simulink model "AntilockBraking"  (R2020b)
settings: Solver=VariableStepAuto  StartTime=0.0  StopTime=10.0  RelTol=1e-3
model workspace (MAT data in the model file):
  I = 5
  Kf = 1
  PBmax = 1500
  Rr = 1.25
  TB = 0.01
  ctrl = 1
  g = 32.18
  h : matlab.ui.Figure (value not decoded)
  m = 50
  mu = [0 0.4 0.8 0.97 1 0.98 0.96 0.94 0.92 0.9 0.88 0.855 0.83 0.81 0.79 0.77 0.75 0.73 0.72 0.71 0.7]
  out = Simulink.SimulationOutput
  out.Data.tout = [0; 0.2; 0.4; 0.6; 0.8; 1; 1.2; 1.4; 1.6; 1.8; 2; 2.2; 2.4; 2.6; 2.8; 3; 3.2; 3.4; 3.6; 3.8; 4; 4.2; 4.4; 4.6; 4.8; 5; 5.2; 5.4; 5.6; 5.8; 6; 6.2; 6.4; 6.6; 6.8; 7; 7.2; 7.4; 7.6; 7.8; 8; 8.2; 8.4; 8.6; 8.8; 9; 9.2; 9.4; 9.6; 9.8; 10]
  out.Data.yout = Simulink.SimulationData.Dataset
  out.Data.yout.any.Name = 'yout'
  out.Data.yout.any.Version = 3
  out.Data.yout.any.Storage = Simulink.SimulationData.Storage.RamDatasetStorage
  out.Data.yout.any.Storage.any.Version = 2
  out.Data.yout.any.Storage.any.Elements{1} = Simulink.SimulationData.Signal
  out.Data.yout.any.Storage.any.Elements{1}.Version = 1
  out.Data.yout.any.Storage.any.Elements{1}.BlockPath = Simulink.SimulationData.BlockPath
  out.Data.yout.any.Storage.any.Elements{1}.BlockPath.path = {'AntilockBraking/Outport1'}
  out.Data.yout.any.Storage.any.Elements{1}.Values = timeseries
  out.Data.yout.any.Storage.any.Elements{1}.Values.Name = 'Ww'
  out.Data.yout.any.Storage.any.Elements{1}.Values.DataInfo = tsdata.datametadata
  out.Data.yout.any.Storage.any.Elements{1}.Values.DataInfo.Interpolation = tsdata.interpolation
  out.Data.yout.any.Storage.any.Elements{1}.Values.DataInfo.Interpolation.Fhandle : function handle (value not decoded)
  out.Data.yout.any.Storage.any.Elements{1}.Values.DataInfo.Interpolation.Name = 'linear'
  out.Data.yout.any.Storage.any.Elements{1}.Values.TimeInfo = tsdata.timemetadata
  out.Data.yout.any.Storage.any.Elements{1}.Values.TimeInfo.Length = 51
  out.Data.yout.any.Storage.any.Elements{1}.Values.TimeInfo.DuplicateTimes = 0
  out.Data.yout.any.Storage.any.Elements{1}.Values.TimeInfo.Time_ = [0; 0.2; 0.4; 0.6; 0.8; 1; 1.2; 1.4; 1.6; 1.8; 2; 2.2; 2.4; 2.6; 2.8; 3; 3.2; 3.4; 3.6; 3.8; 4; 4.2; 4.4; 4.6; 4.8; 5; 5.2; 5.4; 5.6; 5.8; 6; 6.2; 6.4; 6.6; 6.8; 7; 7.2; 7.4; 7.6; 7.8; 8; 8.2; 8.4; 8.6; 8.8; 9; 9.2; 9.4; 9.6; 9.8; 10]
  out.Data.yout.any.Storage.any.Elements{1}.Values.TimeInfo.Initialized = 1
  out.Data.yout.any.Storage.any.Elements{1}.Values.QualityInfo = tsdata.qualmetadata
  out.Data.yout.any.Storage.any.Elements{1}.Values.Data_ = [70.4; 70.4; 70.4; 70.4; 70.4; 70.4; 70.4; 70.4; 70.4; 70.4; 70.4; 70.4; 70.4; 70.4; 70.4; 70.4; 70.4; 70.4; 70.4; 70.4; 70.4; 70.4; 70.4; 70.4; 70.4; 70.4; 70.4; 70.4; 70.4; 70.4; 70.4; 70.4; 70.4; 70.4; 70.4; 70.4; 70.4; 70.4; 70.4; 70.4; 70.4; 70.4; 70.4; 70.4; 70.4; 70.4; 70.4; 70.4; 70.4; 70.4; 70.4]
  out.Data.yout.any.Storage.any.Elements{1}.Name = 'Ww'
  out.Metadata = Simulink.SimulationMetadata
  out.Metadata.ModelInfo.ModelName = 'AntilockBraking'
  out.Metadata.ModelInfo.ModelVersion = '1.2'
  out.Metadata.ModelInfo.ModelFilePath = 'C:\Users\baner\MATLAB\Projects\Problem_3_AntilockBrakingSystem\AntilockBraking.slx'
  out.Metadata.ModelInfo.UserID = 'baner'
  out.Metadata.ModelInfo.MachineName = 'LAPTOP-PBLSD5RN'
  out.Metadata.ModelInfo.Platform = 'PCWIN64'
  out.Metadata.ModelInfo.ModelStructuralChecksum = [3722489804; 3647447735; 815880221; 3047452302]
  out.Metadata.ModelInfo.SimulationMode = 'normal'
  out.Metadata.ModelInfo.StartTime = 0
  out.Metadata.ModelInfo.StopTime = 10
  out.Metadata.ModelInfo.SolverInfo.Type = 'Variable-Step'
  out.Metadata.ModelInfo.SolverInfo.Solver = 'ode45'
  out.Metadata.ModelInfo.SolverInfo.MaxStepSize = 0.2
  out.Metadata.ModelInfo.SimulinkVersion.Name = 'Simulink'
  out.Metadata.ModelInfo.SimulinkVersion.Version = '10.2'
  out.Metadata.ModelInfo.SimulinkVersion.Release = '(R2020b)'
  out.Metadata.ModelInfo.SimulinkVersion.Date = '29-Jul-2020'
  out.Metadata.ModelInfo.LoggingInfo.LoggingToFile = 'off'
  out.Metadata.TimingInfo.WallClockTimestampStart = '2020-12-17 10:27:53'
  out.Metadata.TimingInfo.WallClockTimestampStop = '2020-12-17 10:27:55'
  out.Metadata.TimingInfo.InitializationElapsedWallTime = 1.3877722
  out.Metadata.TimingInfo.ExecutionElapsedWallTime = 0.4189762
  out.Metadata.TimingInfo.TerminationElapsedWallTime = 0.0827791
  out.Metadata.TimingInfo.TotalElapsedWallTime = 1.8895275
  out.Metadata.TimingInfo.ProfilerData = 'Profiler is not enabled'
  out.Metadata.ExecutionInfo.StopEvent = 'ReachedStopTime'
  out.Metadata.ExecutionInfo.StopEventSource = []
  out.Metadata.ExecutionInfo.StopEventDescription = 'Reached stop time of 10'
  out.Metadata.ExecutionInfo.ErrorDiagnostic = []
  out.Metadata.ExecutionInfo.WarningDiagnostics(1).Diagnostic = MSLDiagnostic
  out.Metadata.ExecutionInfo.WarningDiagnostics(1).Diagnostic.identifier = 'Simulink:Engine:MdlFileShadowedByFile'
  out.Metadata.ExecutionInfo.WarningDiagnostics(1).Diagnostic.message = 'The file containing block diagram ''<a href="matlab:open_system (''sldemo_wheelspeed_absbrake'')">sldemo_wheelspeed_absbrake</a>'' is shadowed by a file of the same name higher on the MATLAB path. This can cause unexpected behavior. For more information see <a href="matlab:helpview([docroot ''/toolbox/simulink/helptargets.map''], ''shadowing'')">"Avoiding Problems with Shadowed Files"</a> in the Simulink documentation.
    | 
    | The file containing the block diagram is: C:\Users\baner\OneDrive\Documents\MATLAB\Examples\R2020b\simulink_automotive\ModelingAnAntiLockBrakingSystemExample\sldemo_wheelspeed_absbrake.slx.
    | The file higher on the MATLAB path is: C:\Program Files\MATLAB\R2020b\toolbox\simulink\simdemos\automotive\sldemo_wheelspeed_absbrake.slx'
  out.Metadata.ExecutionInfo.WarningDiagnostics(1).Diagnostic.paths = {'sldemo_wheelspeed_absbrake'}
  out.Metadata.ExecutionInfo.WarningDiagnostics(1).Diagnostic.arguments = {'sldemo_wheelspeed_absbrake', 'C:\Users\baner\OneDrive\Documents\MATLAB\Examples\R2020b\simulink_automotive\ModelingAnAntiLockBrakingSystemExample\sldemo_wheelspeed_absbrake.slx', 'C:\Program Files\MATLAB\R2020b\toolbox\simulink\simdemos\automotive\sldemo_wheelspeed_absbrake.slx'}
  out.Metadata.ExecutionInfo.WarningDiagnostics(1).Diagnostic.stack = struct([])
  out.Metadata.ExecutionInfo.WarningDiagnostics(1).Diagnostic.metaDataProp.UI = []
  out.Metadata.ExecutionInfo.WarningDiagnostics(1).Diagnostic.metaDataProp.STAGE = []
  out.Metadata.ExecutionInfo.WarningDiagnostics(1).Diagnostic.metaDataProp.CATEGORY = []
  out.Metadata.ExecutionInfo.WarningDiagnostics(1).Diagnostic.metaDataProp.COMPONENT = []
  out.Metadata.ExecutionInfo.WarningDiagnostics(1).Diagnostic.metaDataProp.MDL_NAME = []
  out.Metadata.ExecutionInfo.WarningDiagnostics(1).Diagnostic.metaDataProp.ACTION = ''
  out.Metadata.ExecutionInfo.WarningDiagnostics(1).Diagnostic.metaDataProp.DOC = []
  out.Metadata.ExecutionInfo.WarningDiagnostics(1).Diagnostic.metaDataProp.SUB_CATEGORY = []
  out.Metadata.ExecutionInfo.WarningDiagnostics(1).Diagnostic.metaDataProp.MSTACK_PRESERVE = []
  out.Metadata.ExecutionInfo.WarningDiagnostics(1).Diagnostic.metaDataProp.DOUBLE_ARGS = []
  out.Metadata.ExecutionInfo.WarningDiagnostics(1).SimulationPhase = 'Initialization'
  out.Metadata.ExecutionInfo.WarningDiagnostics(1).SimulationTime = []
  out.Metadata.ExecutionInfo.WarningDiagnostics(2).Diagnostic = MSLDiagnostic
  out.Metadata.ExecutionInfo.WarningDiagnostics(2).Diagnostic.identifier = 'Simulink:Engine:MdlFileShadowedByFile'
  out.Metadata.ExecutionInfo.WarningDiagnostics(2).Diagnostic.message = 'The file containing block diagram ''<a href="matlab:open_system (''sldemo_absbrake'')">sldemo_absbrake</a>'' is shadowed by a file of the same name higher on the MATLAB path. This can cause unexpected behavior. For more information see <a href="matlab:helpview([docroot ''/toolbox/simulink/helptargets.map''], ''shadowing'')">"Avoiding Problems with Shadowed Files"</a> in the Simulink documentation.
    | 
    | The file containing the block diagram is: C:\Users\baner\OneDrive\Documents\MATLAB\Examples\R2020b\simulink_automotive\ModelingAnAntiLockBrakingSystemExample\sldemo_absbrake.slx.
    | The file higher on the MATLAB path is: C:\Program Files\MATLAB\R2020b\toolbox\simulink\simdemos\automotive\sldemo_absbrake.slx'
  out.Metadata.ExecutionInfo.WarningDiagnostics(2).Diagnostic.paths = {'sldemo_absbrake'}
  out.Metadata.ExecutionInfo.WarningDiagnostics(2).Diagnostic.arguments = {'sldemo_absbrake', 'C:\Users\baner\OneDrive\Documents\MATLAB\Examples\R2020b\simulink_automotive\ModelingAnAntiLockBrakingSystemExample\sldemo_absbrake.slx', 'C:\Program Files\MATLAB\R2020b\toolbox\simulink\simdemos\automotive\sldemo_absbrake.slx'}
  out.Metadata.ExecutionInfo.WarningDiagnostics(2).Diagnostic.stack = struct([])
  out.Metadata.ExecutionInfo.WarningDiagnostics(2).Diagnostic.metaDataProp.UI = []
  out.Metadata.ExecutionInfo.WarningDiagnostics(2).Diagnostic.metaDataProp.STAGE = []
  out.Metadata.ExecutionInfo.WarningDiagnostics(2).Diagnostic.metaDataProp.CATEGORY = []
  out.Metadata.ExecutionInfo.WarningDiagnostics(2).Diagnostic.metaDataProp.COMPONENT = []
  out.Metadata.ExecutionInfo.WarningDiagnostics(2).Diagnostic.metaDataProp.MDL_NAME = []
  out.Metadata.ExecutionInfo.WarningDiagnostics(2).Diagnostic.metaDataProp.ACTION = ''
  out.Metadata.ExecutionInfo.WarningDiagnostics(2).Diagnostic.metaDataProp.DOC = []
  out.Metadata.ExecutionInfo.WarningDiagnostics(2).Diagnostic.metaDataProp.SUB_CATEGORY = []
  out.Metadata.ExecutionInfo.WarningDiagnostics(2).Diagnostic.metaDataProp.MSTACK_PRESERVE = []
  out.Metadata.ExecutionInfo.WarningDiagnostics(2).Diagnostic.metaDataProp.DOUBLE_ARGS = []
  out.Metadata.ExecutionInfo.WarningDiagnostics(2).SimulationPhase = 'Initialization'
  out.Metadata.ExecutionInfo.WarningDiagnostics(2).SimulationTime = []
  out.Metadata.AppInfo = struct()
  sldemo_absbrake_output = Simulink.SimulationData.Dataset
  sldemo_absbrake_output.any.Name = 'sldemo_absbrake_output'
  sldemo_absbrake_output.any.Version = 3
  sldemo_absbrake_output.any.Storage = Simulink.SimulationData.Storage.RamDatasetStorage
  sldemo_absbrake_output.any.Storage.any.Version = 2
  sldemo_absbrake_output.any.Storage.any.Elements{1} = Simulink.SimulationData.Signal
  sldemo_absbrake_output.any.Storage.any.Elements{1}.PortType = 'outport'
  sldemo_absbrake_output.any.Storage.any.Elements{1}.Version = 1
  sldemo_absbrake_output.any.Storage.any.Elements{1}.BlockPath = Simulink.SimulationData.BlockPath
  sldemo_absbrake_output.any.Storage.any.Elements{1}.BlockPath.path = {'sldemo_absbrake/Bus Creator'}
  sldemo_absbrake_output.any.Storage.any.Elements{1}.Values.Ww = timeseries
  sldemo_absbrake_output.any.Storage.any.Elements{1}.Values.Ww.Name = 'Ww'
  sldemo_absbrake_output.any.Storage.any.Elements{1}.Values.Ww.DataInfo = tsdata.datametadata
  sldemo_absbrake_output.any.Storage.any.Elements{1}.Values.Ww.DataInfo.Interpolation = tsdata.interpolation
  sldemo_absbrake_output.any.Storage.any.Elements{1}.Values.Ww.DataInfo.Interpolation.Fhandle : function handle (value not decoded)
  sldemo_absbrake_output.any.Storage.any.Elements{1}.Values.Ww.DataInfo.Interpolation.Name = 'linear'
  sldemo_absbrake_output.any.Storage.any.Elements{1}.Values.Ww.TimeInfo = tsdata.timemetadata
  sldemo_absbrake_output.any.Storage.any.Elements{1}.Values.Ww.TimeInfo.Length = 1439
  sldemo_absbrake_output.any.Storage.any.Elements{1}.Values.Ww.TimeInfo.DuplicateTimes = 0
  sldemo_absbrake_output.any.Storage.any.Elements{1}.Values.Ww.TimeInfo.Time_ = [0 3.15544362088e-30 2.28353311955e-06 1.37011987173e-05 7.07895267062e-05 0.00035623116665 0.00178343936637 0.00537219040452 0.010890843325 0.0183988159927 0.0278679319875 0.0378679319875 ... (1439 elements, 1439x1)]
  sldemo_absbrake_output.any.Storage.any.Elements{1}.Values.Ww.TimeInfo.Initialized = 1
  sldemo_absbrake_output.any.Storage.any.Elements{1}.Values.Ww.QualityInfo = tsdata.qualmetadata
  sldemo_absbrake_output.any.Storage.any.Elements{1}.Values.Ww.Data_ = [70.4 70.4 70.4 70.4 70.3999999999 70.3999999851 70.3999981998 70.3999552831 70.3996757718 70.3986874337 70.3962654702 70.392251589 ... (1439 elements, 1439x1)]
  sldemo_absbrake_output.any.Storage.any.Elements{1}.Values.Vs = timeseries
  sldemo_absbrake_output.any.Storage.any.Elements{1}.Values.Vs.Name = 'Vs'
  sldemo_absbrake_output.any.Storage.any.Elements{1}.Values.Vs.DataInfo = tsdata.datametadata
  sldemo_absbrake_output.any.Storage.any.Elements{1}.Values.Vs.DataInfo.Interpolation = tsdata.interpolation
  sldemo_absbrake_output.any.Storage.any.Elements{1}.Values.Vs.DataInfo.Interpolation.Fhandle : function handle (value not decoded)
  sldemo_absbrake_output.any.Storage.any.Elements{1}.Values.Vs.DataInfo.Interpolation.Name = 'linear'
  sldemo_absbrake_output.any.Storage.any.Elements{1}.Values.Vs.TimeInfo = tsdata.timemetadata
  sldemo_absbrake_output.any.Storage.any.Elements{1}.Values.Vs.TimeInfo.Length = 1439
  sldemo_absbrake_output.any.Storage.any.Elements{1}.Values.Vs.TimeInfo.DuplicateTimes = 0
  sldemo_absbrake_output.any.Storage.any.Elements{1}.Values.Vs.TimeInfo.Time_ = [0 3.15544362088e-30 2.28353311955e-06 1.37011987173e-05 7.07895267062e-05 0.00035623116665 0.00178343936637 0.00537219040452 0.010890843325 0.0183988159927 0.0278679319875 0.0378679319875 ... (1439 elements, 1439x1)]
  sldemo_absbrake_output.any.Storage.any.Elements{1}.Values.Vs.TimeInfo.Initialized = 1
  sldemo_absbrake_output.any.Storage.any.Elements{1}.Values.Vs.QualityInfo = tsdata.qualmetadata
  sldemo_absbrake_output.any.Storage.any.Elements{1}.Values.Vs.Data_ = [70.4 70.4 70.4 70.4 70.4 70.4 70.3999999994 70.3999999548 70.3999993187 70.3999951932 70.3999785767 70.3999377685 ... (1439 elements, 1439x1)]
  sldemo_absbrake_output.any.Storage.any.Elements{1}.Values.Sd = timeseries
  sldemo_absbrake_output.any.Storage.any.Elements{1}.Values.Sd.Name = 'Sd'
  sldemo_absbrake_output.any.Storage.any.Elements{1}.Values.Sd.DataInfo = tsdata.datametadata
  sldemo_absbrake_output.any.Storage.any.Elements{1}.Values.Sd.DataInfo.Interpolation = tsdata.interpolation
  sldemo_absbrake_output.any.Storage.any.Elements{1}.Values.Sd.DataInfo.Interpolation.Fhandle : function handle (value not decoded)
  sldemo_absbrake_output.any.Storage.any.Elements{1}.Values.Sd.DataInfo.Interpolation.Name = 'linear'
  sldemo_absbrake_output.any.Storage.any.Elements{1}.Values.Sd.TimeInfo = tsdata.timemetadata
  sldemo_absbrake_output.any.Storage.any.Elements{1}.Values.Sd.TimeInfo.Length = 1439
  sldemo_absbrake_output.any.Storage.any.Elements{1}.Values.Sd.TimeInfo.DuplicateTimes = 0
  sldemo_absbrake_output.any.Storage.any.Elements{1}.Values.Sd.TimeInfo.Time_ = [0 3.15544362088e-30 2.28353311955e-06 1.37011987173e-05 7.07895267062e-05 0.00035623116665 0.00178343936637 0.00537219040452 0.010890843325 0.0183988159927 0.0278679319875 0.0378679319875 ... (1439 elements, 1439x1)]
  sldemo_absbrake_output.any.Storage.any.Elements{1}.Values.Sd.TimeInfo.Initialized = 1
  sldemo_absbrake_output.any.Storage.any.Elements{1}.Values.Sd.QualityInfo = tsdata.qualmetadata
  sldemo_absbrake_output.any.Storage.any.Elements{1}.Values.Sd.Data_ = [0 2.77679038638e-28 0.000200950914521 0.00120570548712 0.00622947835014 0.0313483426652 0.15694266424 0.472752755536 0.958394210674 1.6190957839 2.45237785266 3.33237736011 ... (1439 elements, 1439x1)]
  sldemo_absbrake_output.any.Storage.any.Elements{1}.Name = 'yout'
  sldemo_absbrake_output.any.Storage.any.Elements{2} = Simulink.SimulationData.Signal
  sldemo_absbrake_output.any.Storage.any.Elements{2}.PortType = 'outport'
  sldemo_absbrake_output.any.Storage.any.Elements{2}.Version = 1
  sldemo_absbrake_output.any.Storage.any.Elements{2}.BlockPath = Simulink.SimulationData.BlockPath
  sldemo_absbrake_output.any.Storage.any.Elements{2}.BlockPath.path = {'sldemo_absbrake/Relative Slip'}
  sldemo_absbrake_output.any.Storage.any.Elements{2}.Values = timeseries
  sldemo_absbrake_output.any.Storage.any.Elements{2}.Values.Name = 'slp'
  sldemo_absbrake_output.any.Storage.any.Elements{2}.Values.DataInfo = tsdata.datametadata
  sldemo_absbrake_output.any.Storage.any.Elements{2}.Values.DataInfo.Interpolation = tsdata.interpolation
  sldemo_absbrake_output.any.Storage.any.Elements{2}.Values.DataInfo.Interpolation.Fhandle : function handle (value not decoded)
  sldemo_absbrake_output.any.Storage.any.Elements{2}.Values.DataInfo.Interpolation.Name = 'linear'
  sldemo_absbrake_output.any.Storage.any.Elements{2}.Values.TimeInfo = tsdata.timemetadata
  sldemo_absbrake_output.any.Storage.any.Elements{2}.Values.TimeInfo.Length = 1439
  sldemo_absbrake_output.any.Storage.any.Elements{2}.Values.TimeInfo.DuplicateTimes = 0
  sldemo_absbrake_output.any.Storage.any.Elements{2}.Values.TimeInfo.Time_ = [0 3.15544362088e-30 2.28353311955e-06 1.37011987173e-05 7.07895267062e-05 0.00035623116665 0.00178343936637 0.00537219040452 0.010890843325 0.0183988159927 0.0278679319875 0.0378679319875 ... (1439 elements, 1439x1)]
  sldemo_absbrake_output.any.Storage.any.Elements{2}.Values.TimeInfo.Initialized = 1
  sldemo_absbrake_output.any.Storage.any.Elements{2}.Values.QualityInfo = tsdata.qualmetadata
  sldemo_absbrake_output.any.Storage.any.Elements{2}.Values.Data_ = [0 0 0 1.21014309684e-14 1.67621472258e-12 2.11920592186e-10 2.55623952006e-08 6.3454228616e-07 4.59583624723e-06 1.85761311049e-05 5.2743005722e-05 0.000109178782748 ... (1439 elements, 1439x1)]
  sldemo_absbrake_output.any.Storage.any.Elements{2}.Name = 'slp'
  slip = [0 0.05 0.1 0.15 0.2 0.25 0.3 0.35 0.4 0.45 0.5 0.55 0.6 0.65 0.7 0.75 0.8 0.85 0.9 0.95 1]
  v0 = 88
settings Model: Creator=baner  LastModifiedBy=baner

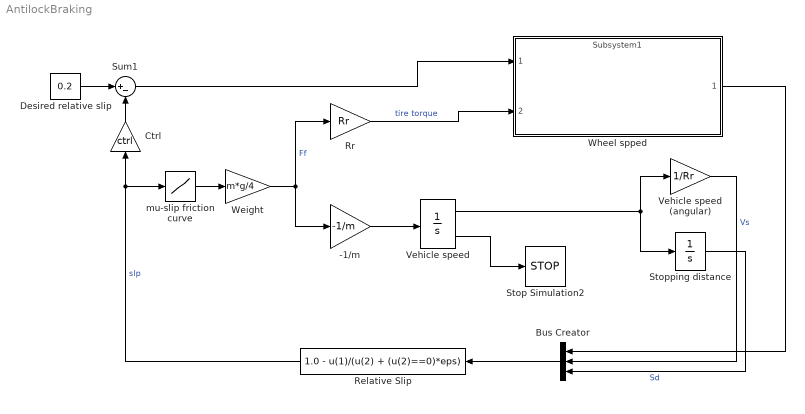
== system AntilockBraking ==
  -1/m : Gain  Gain=-1/m  SaturateOnIntegerOverflow=on  OutDataTypeStr=Inherit: Same as input  ParamDataTypeStr=Inherit: Same as input
  Bus Creator : BusCreator  Inputs=3
  Ctrl : Gain  Gain=ctrl  SaturateOnIntegerOverflow=on  OutDataTypeStr=Inherit: Same as input  ParamDataTypeStr=Inherit: Same as input
  Desired relative slip : Constant  Value=0.2
  Relative Slip : Fcn  Expr=1.0 - u(1)/(u(2) + (u(2)==0)*eps)
  Rr : Gain  Gain=Rr  SaturateOnIntegerOverflow=on  OutDataTypeStr=Inherit: Same as input  ParamDataTypeStr=Inherit: Same as input
  Stop Simulation2 : Stop
  Stopping distance : Integrator  UpperSaturationLimit=1000  LowerSaturationLimit=0
  Sum1 : Sum  Inputs=|+-  InputSameDT=on  SaturateOnIntegerOverflow=on  OutDataTypeStr=Inherit: Same as first input
  Vehicle speed : Integrator  InitialCondition=v0  LimitOutput=on  UpperSaturationLimit=1000  LowerSaturationLimit=0  ShowSaturationPort=on
  Vehicle speed (angular) : Gain  Gain=1/Rr  SaturateOnIntegerOverflow=on  OutDataTypeStr=Inherit: Same as input  ParamDataTypeStr=Inherit: Same as input
  Weight : Gain  Gain=m*g/4  SaturateOnIntegerOverflow=on  OutDataTypeStr=Inherit: Same as input  ParamDataTypeStr=Inherit: Same as input
  Wheel spped : ModelReference  ModelNameDialog=Subsystem1  SimulationMode=Normal  ModelReferenceVersion=1.5
  mu-slip friction curve : Lookup_n-D  NumberOfTableDimensions=1  BreakpointsForDimension1=slip  Table=mu  SaturateOnIntegerOverflow=on  InputSameDT=on
  wires:
  Rr/1 -> Wheel spped/2  "tire torque"
  Sum1/1 -> Wheel spped/1
  Desired relative slip/1 -> Sum1/1
  Ctrl/1 -> Sum1/2
  Weight/1 -> Rr/1, -1/m/1  "Ff"
  mu-slip friction curve/1 -> Weight/1
  -1/m/1 -> Vehicle speed/1
  Relative Slip/1 -> Ctrl/1, mu-slip friction curve/1  "slp"
  Vehicle speed/1 -> Vehicle speed (angular)/1, Stopping distance/1
  Vehicle speed/2 -> Stop Simulation2/1
  Bus Creator/1 -> Relative Slip/1
  Wheel spped/1 -> Bus Creator/1
  Vehicle speed (angular)/1 -> Bus Creator/2  "Vs"
  Stopping distance/1 -> Bus Creator/3  "Sd"
